simulink model "sim3"  (R2023b)
settings: Solver=VariableStepAuto  StartTime=0.0  StopTime=365  RelTol=1e-3
settings Model: Creator=denismatveev  LastModifiedBy=denismatveev

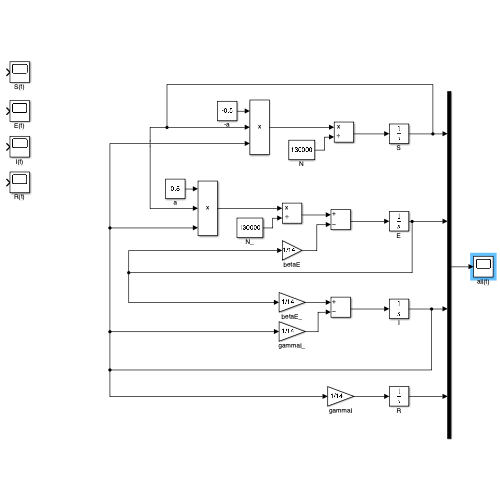
[thumbnail: Simulink's stored preview of the top-level diagram]
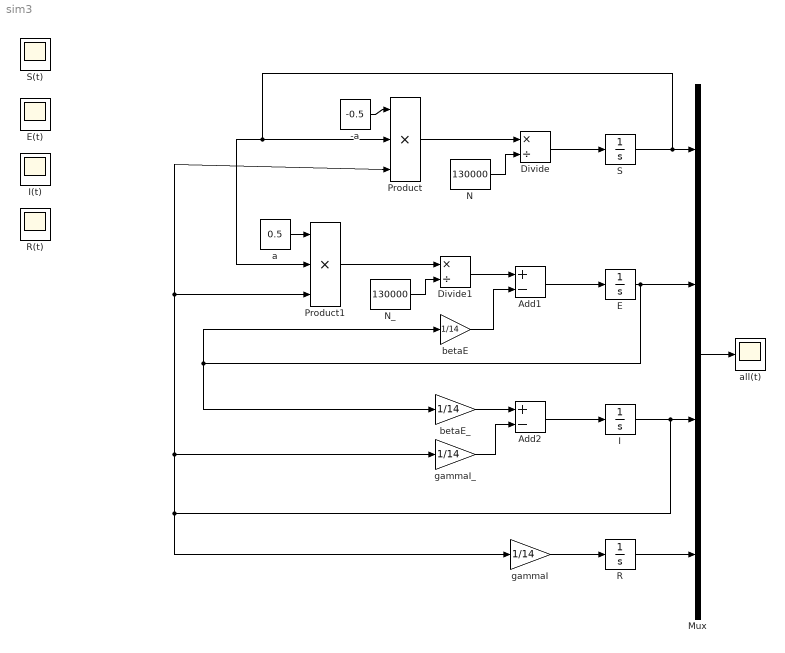
== system sim3 ==
  -a : Constant  Value=-0.5
  Add1 : Sum  Inputs=+-
  Add2 : Sum  Inputs=+-
  Divide : Product  Inputs=*/
  Divide1 : Product  Inputs=*/
  E : Integrator  InitialCondition=3000
  E(t) : Scope
  I : Integrator  InitialCondition=6000
  I(t) : Scope
  Mux : Mux
  N : Constant  Value=130000
  N_ : Constant  Value=130000
  Product : Product  Inputs=3
  Product1 : Product  Inputs=3
  R : Integrator
  R(t) : Scope
  S : Integrator  InitialCondition=121000
  S(t) : Scope
  a : Constant  Value=0.5
  all(t) : Scope
  betaE : Gain  Gain=1/14
  betaE_ : Gain  Gain=1/14
  gammaI : Gain  Gain=1/14
  gammaI_ : Gain  Gain=1/14
  wires:
  S/1 -> Product/2, Product1/2, Mux/1
  -a/1 -> Product/1
  N/1 -> Divide/2
  Product/1 -> Divide/1
  Divide/1 -> S/1
  a/1 -> Product1/1
  Product1/1 -> Divide1/1
  N_/1 -> Divide1/2
  Divide1/1 -> Add1/1
  Add1/1 -> E/1
  E/1 -> Mux/2, betaE_/1, betaE/1
  betaE/1 -> Add1/2
  I/1 -> gammaI/1, gammaI_/1, Product/3, Product1/3, Mux/3
  Add2/1 -> I/1
  betaE_/1 -> Add2/1
  gammaI_/1 -> Add2/2
  gammaI/1 -> R/1
  R/1 -> Mux/4
  Mux/1 -> all(t)/1
